simulink model "MGDC_COMPARACION"  (R2025b)
settings: Solver=VariableStepAuto  StartTime=0.0  StopTime=12  RelTol=1e-3
libraries: spsGroundLib x16, spsSeriesRLCBranchLib x7, spsControlledVoltageSourceLib x6, spsCurrentMeasurementLib x6, spsVoltageMeasurementLib x6, slpidlib x3, spsParallelRLCBranchLib x3, spsBreakerLib x2, sps_lib x1
(part 1 of 4)
settings Model: Creator=joseA  LastModifiedBy=joseA

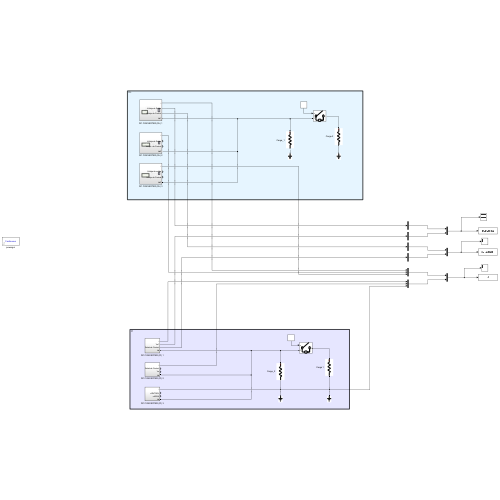
[thumbnail: Simulink's stored preview of the top-level diagram]
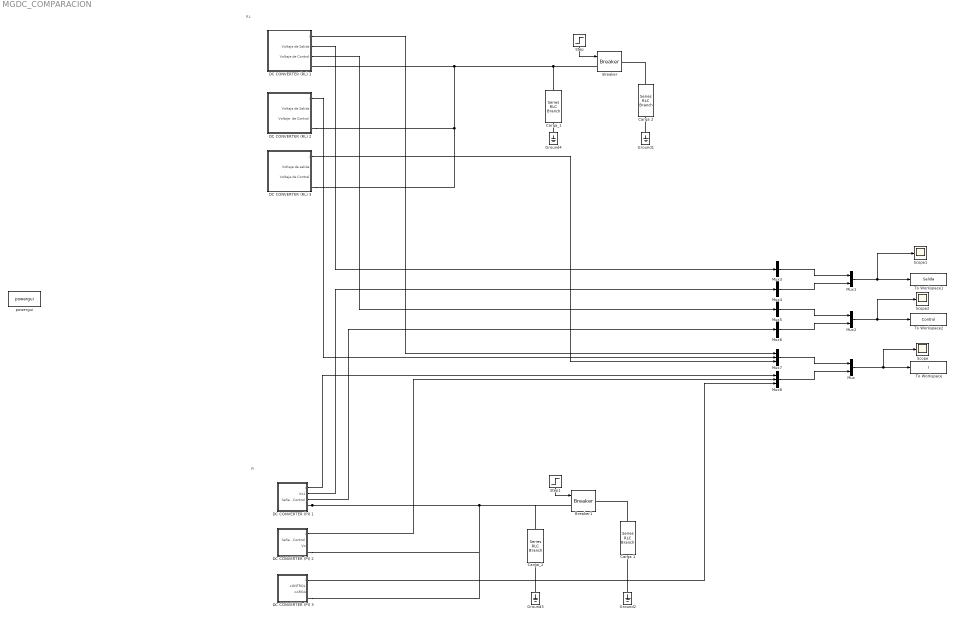
== system MGDC_COMPARACION ==
  note: RL
  note: PI
  Breaker : spsBreakerLib/Breaker  InitialState=0  SwitchingTimes="[1/60  5/60]"  External=on  BreakerResistance=0.01  SnubberResistance=1e6  SnubberCapacitance=inf  Measurements=None  MoreParameters=on  NoBreakLoop=off
  Breaker1 : spsBreakerLib/Breaker  InitialState=0  SwitchingTimes="[1/60  5/60]"  External=on  BreakerResistance=0.01  SnubberResistance=1e6  SnubberCapacitance=inf  Measurements=None  MoreParameters=on  NoBreakLoop=off
  Carga 1 : spsSeriesRLCBranchLib/Series RLC Branch  LConnTagsString=__new0  RConnTagsString=__new0  BranchType=R  Resistance=4  Inductance=1e-3  SetiL0=off  InitialCurrent=0  Capacitance=1e-6  Setx0=off  InitialVoltage=0  Measurements=None
  Carga 2 : spsSeriesRLCBranchLib/Series RLC Branch  LConnTagsString=__new0  RConnTagsString=__new0  BranchType=R  Resistance=4  Inductance=1e-3  SetiL0=off  InitialCurrent=0  Capacitance=1e-6  Setx0=off  InitialVoltage=0  Measurements=None
  Carga_1 : spsSeriesRLCBranchLib/Series RLC Branch  LConnTagsString=__new0  RConnTagsString=__new0  BranchType=R  Resistance=8  Inductance=1e-3  SetiL0=off  InitialCurrent=0  Capacitance=1e-6  Setx0=off  InitialVoltage=0  Measurements=None
  Carga_2 : spsSeriesRLCBranchLib/Series RLC Branch  LConnTagsString=__new0  RConnTagsString=__new0  BranchType=R  Resistance=8  Inductance=1e-3  SetiL0=off  InitialCurrent=0  Capacitance=1e-6  Setx0=off  InitialVoltage=0  Measurements=None
  DC CONVERTER (PI) 1 : Subsystem
      settings: PortSchema="{\"entries\":[{\"content\":{\"sides\":[{\"content\":{\"connectorIds\":[\"Out1\",\"Out2\",\"Out3\",\"LConn1\"]},\"type\":\"ConnectorPlacement.EquallySpacedRectSide\",\"uuid\":\"35976870-9b6d-41fa-84c3-6a07a84f2598\"},{\"content\":{\"side\":\"RIGHT\"},\"type\":\"ConnectorPlacement.EquallySpacedRectSide\",\"uuid\":\"2aca6fb9-572f-479a-9834-ebae41799751\"},{\"content\":{\"side\":\"TOP\"},\"type\":\"ConnectorPlacement.EquallySpacedRectSide\",\"uuid\":\"9763f1a6-ce88-4779-87cd-07f32833b3c9\"}]},\"type\":\"ConnectorPlacement.EquallySpacedConnector\",\"uuid\":\"787491d0-6cf4-4606-8410-63a22802da97\"}],\"packageUris\":[\"http://schema.mathworks.com/mf0/Connector/R2020b\"],\"version\":\"1.0\"}"
  DC CONVERTER (PI) 2 : Subsystem
      settings: PortSchema="{\"entries\":[{\"content\":{\"sides\":[{\"content\":{\"connectorIds\":[\"Out1\",\"Out2\",\"Out3\",\"LConn1\"]},\"type\":\"ConnectorPlacement.EquallySpacedRectSide\",\"uuid\":\"35976870-9b6d-41fa-84c3-6a07a84f2598\"},{\"content\":{\"side\":\"RIGHT\"},\"type\":\"ConnectorPlacement.EquallySpacedRectSide\",\"uuid\":\"2aca6fb9-572f-479a-9834-ebae41799751\"},{\"content\":{\"side\":\"TOP\"},\"type\":\"ConnectorPlacement.EquallySpacedRectSide\",\"uuid\":\"9763f1a6-ce88-4779-87cd-07f32833b3c9\"}]},\"type\":\"ConnectorPlacement.EquallySpacedConnector\",\"uuid\":\"787491d0-6cf4-4606-8410-63a22802da97\"}],\"packageUris\":[\"http://schema.mathworks.com/mf0/Connector/R2020b\"],\"version\":\"1.0\"}"
  DC CONVERTER (PI) 3 : Subsystem
      settings: PortSchema="{\"entries\":[{\"content\":{\"sides\":[{\"content\":{\"connectorIds\":[\"Out1\",\"Out2\",\"Out3\",\"LConn1\"]},\"type\":\"ConnectorPlacement.EquallySpacedRectSide\",\"uuid\":\"35976870-9b6d-41fa-84c3-6a07a84f2598\"},{\"content\":{\"side\":\"RIGHT\"},\"type\":\"ConnectorPlacement.EquallySpacedRectSide\",\"uuid\":\"2aca6fb9-572f-479a-9834-ebae41799751\"},{\"content\":{\"side\":\"TOP\"},\"type\":\"ConnectorPlacement.EquallySpacedRectSide\",\"uuid\":\"9763f1a6-ce88-4779-87cd-07f32833b3c9\"}]},\"type\":\"ConnectorPlacement.EquallySpacedConnector\",\"uuid\":\"787491d0-6cf4-4606-8410-63a22802da97\"}],\"packageUris\":[\"http://schema.mathworks.com/mf0/Connector/R2020b\"],\"version\":\"1.0\"}"
  DC CONVERTER (RL) 1 : Subsystem
      settings: PortSchema="{\"entries\":[{\"content\":{\"sides\":[{\"content\":{\"connectorIds\":[\"Out1\",\"Out2\",\"Out3\",\"LConn1\"]},\"type\":\"ConnectorPlacement.EquallySpacedRectSide\",\"uuid\":\"ef85fad9-e9fc-446c-84f1-0628c69dc682\"},{\"content\":{\"side\":\"RIGHT\"},\"type\":\"ConnectorPlacement.EquallySpacedRectSide\",\"uuid\":\"b40e7fcd-3dee-4863-8a64-1e7c5a18af7f\"},{\"content\":{\"side\":\"TOP\"},\"type\":\"ConnectorPlacement.EquallySpacedRectSide\",\"uuid\":\"d80d7a5f-fa61-4dc2-bf12-1a6ce1f92f0b\"}]},\"type\":\"ConnectorPlacement.EquallySpacedConnector\",\"uuid\":\"ea08e065-469c-42e9-9976-17e3ee08db16\"}],\"packageUris\":[\"http://schema.mathworks.com/mf0/Connector/R2020b\"],\"version\":\"1.0\"}"
  DC CONVERTER (RL) 2 : Subsystem
      settings: PortSchema="{\"entries\":[{\"content\":{\"sides\":[{\"content\":{\"connectorIds\":[\"Out1\",\"Out2\",\"Out3\",\"LConn1\"]},\"type\":\"ConnectorPlacement.EquallySpacedRectSide\",\"uuid\":\"ef85fad9-e9fc-446c-84f1-0628c69dc682\"},{\"content\":{\"side\":\"RIGHT\"},\"type\":\"ConnectorPlacement.EquallySpacedRectSide\",\"uuid\":\"b40e7fcd-3dee-4863-8a64-1e7c5a18af7f\"},{\"content\":{\"side\":\"TOP\"},\"type\":\"ConnectorPlacement.EquallySpacedRectSide\",\"uuid\":\"d80d7a5f-fa61-4dc2-bf12-1a6ce1f92f0b\"}]},\"type\":\"ConnectorPlacement.EquallySpacedConnector\",\"uuid\":\"ea08e065-469c-42e9-9976-17e3ee08db16\"}],\"packageUris\":[\"http://schema.mathworks.com/mf0/Connector/R2020b\"],\"version\":\"1.0\"}"
  DC CONVERTER (RL) 3 : Subsystem
      settings: PortSchema="{\"entries\":[{\"content\":{\"sides\":[{\"content\":{\"connectorIds\":[\"Out1\",\"Out2\",\"Out3\",\"LConn1\"]},\"type\":\"ConnectorPlacement.EquallySpacedRectSide\",\"uuid\":\"ef85fad9-e9fc-446c-84f1-0628c69dc682\"},{\"content\":{\"side\":\"RIGHT\"},\"type\":\"ConnectorPlacement.EquallySpacedRectSide\",\"uuid\":\"b40e7fcd-3dee-4863-8a64-1e7c5a18af7f\"},{\"content\":{\"side\":\"TOP\"},\"type\":\"ConnectorPlacement.EquallySpacedRectSide\",\"uuid\":\"d80d7a5f-fa61-4dc2-bf12-1a6ce1f92f0b\"}]},\"type\":\"ConnectorPlacement.EquallySpacedConnector\",\"uuid\":\"ea08e065-469c-42e9-9976-17e3ee08db16\"}],\"packageUris\":[\"http://schema.mathworks.com/mf0/Connector/R2020b\"],\"version\":\"1.0\"}"
  Ground{1..4} (4 alike) : spsGroundLib/Ground  LConnTagsString=a
  Mux : Mux  Inputs=2
  Mux1 : Mux  Inputs=2
  Mux2 : Mux  Inputs=2
  Mux{3..6} (4 alike) : Mux  Inputs=1
  Mux7 : Mux  Inputs=3
  Mux8 : Mux  Inputs=3
  Scope : Scope
      settings: ActiveDisplayYMinimum=-0.45527999273700881  ActiveDisplayYMaximum=4.74994391053149
  Scope1 : Scope
      settings: ActiveDisplayYMinimum=21.795935750117668  ActiveDisplayYMaximum=24.098400490338538  DataLoggingVariableName=ScopeData4
  Scope2 : Scope
      settings: ActiveDisplayYMinimum=-3.0400673086386818  ActiveDisplayYMaximum=27.410605777748142  DataLoggingVariableName=ScopeData2
  Step : Step  Time=6.5  SampleTime=0
  Step1 : Step  Time=6.5  SampleTime=0
  To Workspace : ToWorkspace  VariableName=I  SaveFormat=Timeseries  SampleTime=-1
  To Workspace1 : ToWorkspace  VariableName=Salida  SaveFormat=Timeseries  SampleTime=-1
  To Workspace2 : ToWorkspace  VariableName=Control  SaveFormat=Timeseries  SampleTime=-1
  powergui : sps_lib/powergui  Priority=1  SimulationMode=Continuous  SampleTime=50e-6  frequency=60  Iterations=50  frequencyindice=0  Pbase=100e6  ErrMax=1e-4  UnitsV=kV  UnitsW=MW  buscounter=0  FunctionMessages=off  echomessages=off  EnableUseOfTLC=off  CurrentSourceSwitches=off  DisableSnubberDevices=off  DisableRonSwitches=off  DisableVfSwitches=off  DisplayEquations=off  AutomaticDiscreteSolvers=off  SolverType=Tustin/Backward Euler (TBE)  Interpol=off  ExternalGateDelay=off  methode=off  Ts=100  x0status=blocks  SPID=on  SwTol=0  HookPort=off  NonlinearTolerance=1e-4  nMaxIteration=100  ContinueOnMaxIteration=off  RestoreLinks=warning  ResistiveCurrentMeasurement=off  Frange=[0:2:500]  Ylog=off  Xlog=on  ShowGrid=off  save=off  variable=ZData  structure=0  ZoomFFT=off  StartTime=0.0  cycles=1  DisplayStyle=1  fundamental=60  FreqAxis=off  MaxFrequency=1000  frequencyindicesteady=1  RmsSteady=1  display=off
  wires:
  DC CONVERTER (PI) 1/3(Señal de Control) -> Mux6/1
  DC CONVERTER (PI) 1/1(i) -> Mux8/1
  Mux5/1 -> Mux2/1
  Mux7/1 -> Mux/1
  Mux3/1 -> Mux1/1
  DC CONVERTER (PI) 1/2(Vo1) -> Mux4/1
  Mux4/1 -> Mux1/2
  DC CONVERTER (PI) 2/1(i) -> Mux8/2
  Mux6/1 -> Mux2/2
  DC CONVERTER (RL) 1/3(Voltaje de Control) -> Mux5/1
  DC CONVERTER (RL) 1/1(i) -> Mux7/1
  DC CONVERTER (RL) 1/2(Voltaje de Salida) -> Mux3/1
  Mux2/1 -> Scope2/1, To Workspace2/1
  Step/1 -> Breaker/1
  Mux/1 -> To Workspace/1, Scope/1
  DC CONVERTER (PI) 3/1(i) -> Mux8/3
  Mux8/1 -> Mux/2
  Mux1/1 -> To Workspace1/1, Scope1/1
  DC CONVERTER (RL) 3/1(i) -> Mux7/3
  Step1/1 -> Breaker1/1
  DC CONVERTER (RL) 2/1(i) -> Mux7/2
  connections:
  DC CONVERTER (PI) 1/LConn1 -- Breaker1/LConn1 -- Carga_2/LConn1 -- DC CONVERTER (PI) 3/LConn1 -- DC CONVERTER (PI) 2/LConn1
  DC CONVERTER (RL) 3/LConn1 -- DC CONVERTER (RL) 2/LConn1 -- Breaker/LConn1 -- Carga_1/LConn1 -- DC CONVERTER (RL) 1/LConn1
  Carga 1/LConn1 -- Breaker1/RConn1
  Ground1/LConn1 -- Carga 2/RConn1
  Ground3/LConn1 -- Carga_2/RConn1
  Ground2/LConn1 -- Carga 1/RConn1
  Ground4/LConn1 -- Carga_1/RConn1
  Carga 2/LConn1 -- Breaker/RConn1

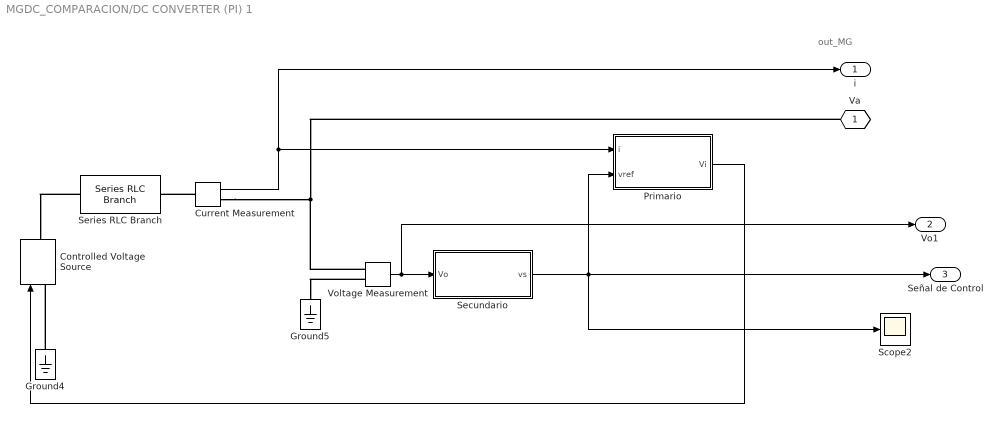
== system MGDC_COMPARACION/DC CONVERTER (PI) 1 ==
  note: out_MG
  Controlled Voltage Source : spsControlledVoltageSourceLib/Controlled Voltage Source  Initialize=on  Source_Type=DC  Amplitude=0  Phase=0  Frequency=0  Measurements=None
  Current Measurement : spsCurrentMeasurementLib/Current Measurement  PhasorSimulation=off  OutputType=Complex  PSBequivalent=0
  Ground4 : spsGroundLib/Ground  LConnTagsString=a
  Ground5 : spsGroundLib/Ground  LConnTagsString=a
  Primario : Subsystem
  Scope2 : Scope
      settings: ActiveDisplayYMinimum=21.641164987150439  ActiveDisplayYMaximum=24.237473255707151  DataLoggingVariableName=ScopeData3
  Secundario : Subsystem
  Series RLC Branch : spsSeriesRLCBranchLib/Series RLC Branch  LConnTagsString=__new0  RConnTagsString=__new0  BranchType=R  Resistance=0.1  Inductance=1e-3  SetiL0=off  InitialCurrent=0  Capacitance=1e-6  Setx0=off  InitialVoltage=0  Measurements=None
  Voltage Measurement : spsVoltageMeasurementLib/Voltage Measurement  PhasorSimulation=off  OutputType=Complex  PSBequivalent=0
  Va : PMIOPort  Tag=PMCPort  Side=Left
  i : Outport
  Vo1 : Outport  Port=2
  Señal de Control : Outport  Port=3
  wires:
  Voltage Measurement/1 -> Vo1/1, Secundario/1(Vo)
  Current Measurement/1 -> i/1, Primario/1(i)
  Secundario/1(vs) -> Primario/2(vref), Señal de Control/1, Scope2/1
  Primario/1(Vi) -> Controlled Voltage Source/1
  connections:
  Series RLC Branch/LConn1 -- Controlled Voltage Source/RConn1
  Ground4/LConn1 -- Controlled Voltage Source/LConn1
  Current Measurement/LConn1 -- Series RLC Branch/RConn1
  Current Measurement/RConn1 -- Voltage Measurement/LConn1 -- Va/RConn1
  Voltage Measurement/LConn2 -- Ground5/LConn1

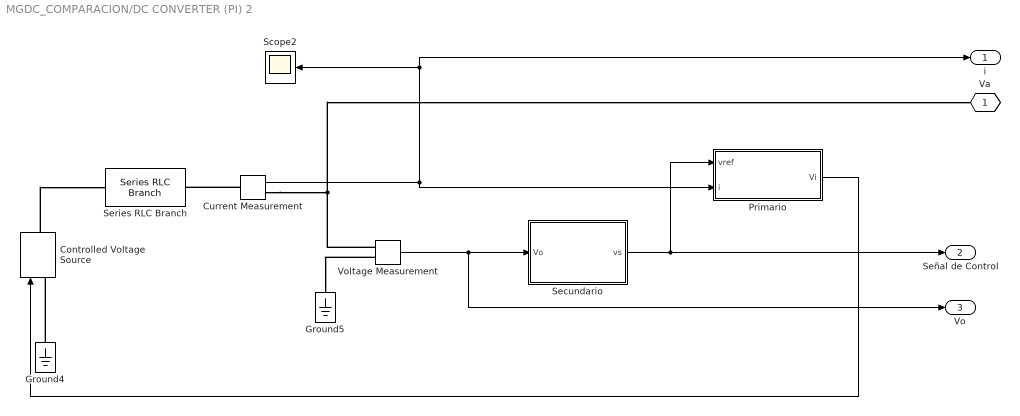
== system MGDC_COMPARACION/DC CONVERTER (PI) 2 ==
  Controlled Voltage Source : spsControlledVoltageSourceLib/Controlled Voltage Source  Initialize=on  Source_Type=DC  Amplitude=0  Phase=0  Frequency=0  Measurements=None
  Current Measurement : spsCurrentMeasurementLib/Current Measurement  PhasorSimulation=off  OutputType=Complex  PSBequivalent=0
  Ground4 : spsGroundLib/Ground  LConnTagsString=a
  Ground5 : spsGroundLib/Ground  LConnTagsString=a
  Primario : Subsystem
  Scope2 : Scope
      settings: ActiveDisplayYMinimum=26.65957  ActiveDisplayYMaximum=30.33414
  Secundario : Subsystem
  Series RLC Branch : spsSeriesRLCBranchLib/Series RLC Branch  LConnTagsString=__new0  RConnTagsString=__new0  BranchType=R  Resistance=0.1  Inductance=1e-3  SetiL0=off  InitialCurrent=0  Capacitance=1e-6  Setx0=off  InitialVoltage=0  Measurements=None
  Voltage Measurement : spsVoltageMeasurementLib/Voltage Measurement  PhasorSimulation=off  OutputType=Complex  PSBequivalent=0
  Va : PMIOPort  Tag=PMCPort  Side=Left
  i : Outport
  Señal de Control : Outport  Port=2
  Vo : Outport  Port=3
  wires:
  Primario/1(Vi) -> Controlled Voltage Source/1
  Secundario/1(vs) -> Primario/1(vref), Señal de Control/1
  Current Measurement/1 -> i/1, Scope2/1, Primario/2(i)
  Voltage Measurement/1 -> Vo/1, Secundario/1(Vo)
  connections:
  Voltage Measurement/LConn2 -- Ground5/LConn1
  Voltage Measurement/LConn1 -- Va/RConn1 -- Current Measurement/RConn1
  Current Measurement/LConn1 -- Series RLC Branch/RConn1
  Ground4/LConn1 -- Controlled Voltage Source/LConn1
  Controlled Voltage Source/RConn1 -- Series RLC Branch/LConn1

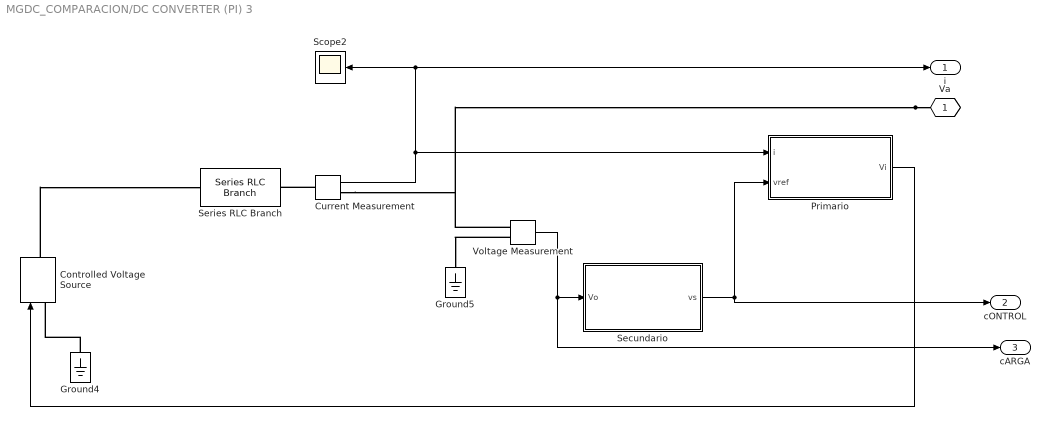
== system MGDC_COMPARACION/DC CONVERTER (PI) 3 ==
  Controlled Voltage Source : spsControlledVoltageSourceLib/Controlled Voltage Source  Initialize=on  Source_Type=DC  Amplitude=0  Phase=0  Frequency=0  Measurements=None
  Current Measurement : spsCurrentMeasurementLib/Current Measurement  PhasorSimulation=off  OutputType=Complex  PSBequivalent=0
  Ground4 : spsGroundLib/Ground  LConnTagsString=a
  Ground5 : spsGroundLib/Ground  LConnTagsString=a
  Primario : Subsystem
  Scope2 : Scope
      settings: ActiveDisplayYMinimum=-2.79721  ActiveDisplayYMaximum=25.17493
  Secundario : Subsystem
  Series RLC Branch : spsSeriesRLCBranchLib/Series RLC Branch  LConnTagsString=__new0  RConnTagsString=__new0  BranchType=R  Resistance=0.1  Inductance=1e-3  SetiL0=off  InitialCurrent=0  Capacitance=1e-6  Setx0=off  InitialVoltage=0  Measurements=None
  Voltage Measurement : spsVoltageMeasurementLib/Voltage Measurement  PhasorSimulation=off  OutputType=Complex  PSBequivalent=0
  Va : PMIOPort  Tag=PMCPort  Side=Left
  i : Outport
  cONTROL : Outport  Port=2
  cARGA : Outport  Port=3
  wires:
  Primario/1(Vi) -> Controlled Voltage Source/1
  Secundario/1(vs) -> cONTROL/1, Primario/2(vref)
  Current Measurement/1 -> i/1, Scope2/1, Primario/1(i)
  Voltage Measurement/1 -> cARGA/1, Secundario/1(Vo)
  connections:
  Controlled Voltage Source/RConn1 -- Series RLC Branch/LConn1
  Voltage Measurement/LConn2 -- Ground5/LConn1
  Va/RConn1 -- Voltage Measurement/LConn1 -- Current Measurement/RConn1
  Current Measurement/LConn1 -- Series RLC Branch/RConn1
  Ground4/LConn1 -- Controlled Voltage Source/LConn1

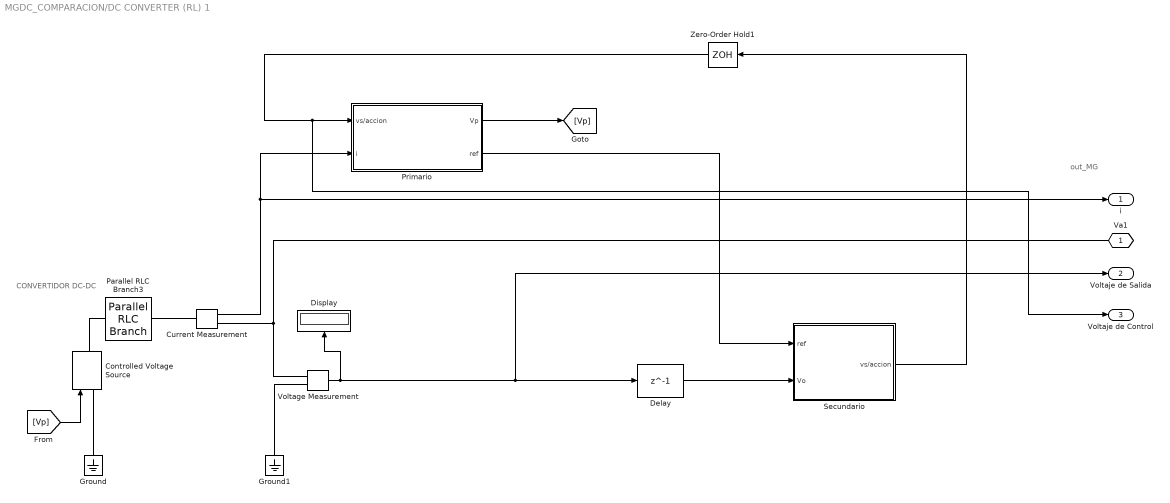
== system MGDC_COMPARACION/DC CONVERTER (RL) 1 ==
  note: out_MG
  note: CONVERTIDOR DC-DC
  Controlled Voltage Source : spsControlledVoltageSourceLib/Controlled Voltage Source  Initialize=on  Source_Type=DC  Amplitude=0  Phase=0  Frequency=0  Measurements=None
  Current Measurement : spsCurrentMeasurementLib/Current Measurement  PhasorSimulation=off  OutputType=Complex  PSBequivalent=0
  Delay : Delay  DelayLength=1  InitialCondition=0  UseCircularBuffer=on
  Display : Display
  Ground : spsGroundLib/Ground  LConnTagsString=a
  Ground1 : spsGroundLib/Ground  LConnTagsString=a
  Parallel RLC Branch3 : spsParallelRLCBranchLib/Parallel RLC Branch  LConnTagsString=a  RConnTagsString=__new0  BranchType=R  Resistance=0.01  Inductance=1e-3  SetiL0=off  InitialCurrent=0  Capacitance=1e-6  Setx0=off  InitialVoltage=0  Measurements=None
  Primario : Subsystem
  "Secundario " : Subsystem
  Voltage Measurement : spsVoltageMeasurementLib/Voltage Measurement  PhasorSimulation=off  OutputType=Complex  PSBequivalent=0
  Zero-Order Hold1 : ZeroOrderHold  SampleTime=0.01
  Va1 : PMIOPort  Tag=PMCPort  Side=Left
  i : Outport
  Voltaje de Salida : Outport  Port=2
  Voltaje de Control : Outport  Port=3
  wires:
  Voltage Measurement/1 -> Voltaje de Salida/1, Delay/1, Display/1
  [Vp] -> Controlled Voltage Source/1
  Zero-Order Hold1/1 -> Voltaje de Control/1, Primario/1(vs/accion)
  Current Measurement/1 -> i/1, Primario/2(i)
  "Secundario "/1(vs/accion) -> Zero-Order Hold1/1
  Primario/2(ref) -> "Secundario "/1(ref)
  Delay/1 -> "Secundario "/2(Vo)
  Primario/1(Vp) -> [Vp]
  connections:
  Voltage Measurement/LConn2 -- Ground1/LConn1
  Ground/LConn1 -- Controlled Voltage Source/LConn1
  Parallel RLC Branch3/LConn1 -- Current Measurement/LConn1
  Voltage Measurement/LConn1 -- Va1/RConn1 -- Current Measurement/RConn1
  Controlled Voltage Source/RConn1 -- Parallel RLC Branch3/RConn1

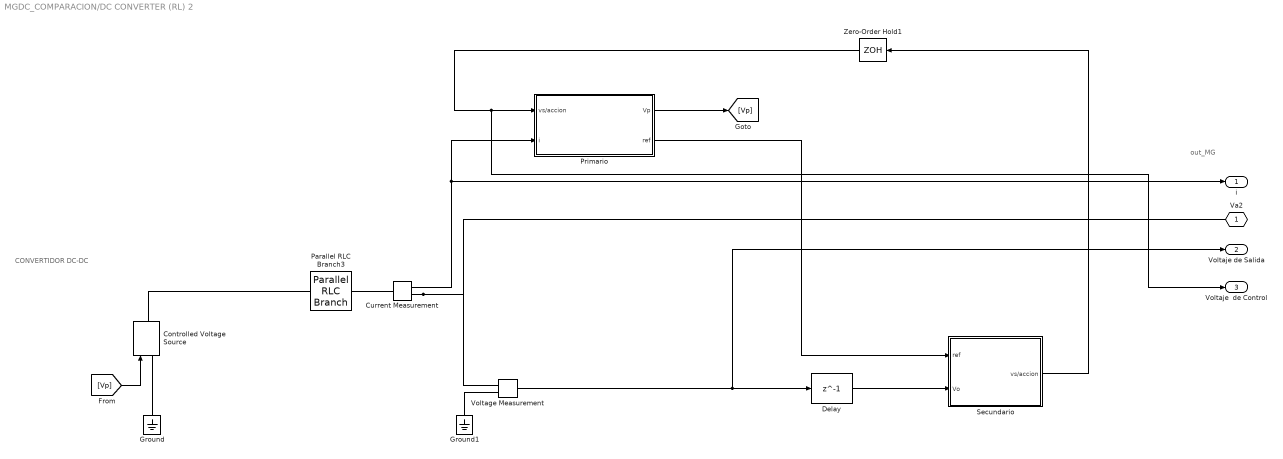
== system MGDC_COMPARACION/DC CONVERTER (RL) 2 ==
  note: out_MG
  note: CONVERTIDOR DC-DC
  Controlled Voltage Source : spsControlledVoltageSourceLib/Controlled Voltage Source  Initialize=on  Source_Type=DC  Amplitude=0  Phase=0  Frequency=0  Measurements=None
  Current Measurement : spsCurrentMeasurementLib/Current Measurement  PhasorSimulation=off  OutputType=Complex  PSBequivalent=0
  Delay : Delay  DelayLength=1  InitialCondition=0  UseCircularBuffer=on
  Ground : spsGroundLib/Ground  LConnTagsString=a
  Ground1 : spsGroundLib/Ground  LConnTagsString=a
  Parallel RLC Branch3 : spsParallelRLCBranchLib/Parallel RLC Branch  LConnTagsString=a  RConnTagsString=__new0  BranchType=R  Resistance=0.01  Inductance=1e-3  SetiL0=off  InitialCurrent=0  Capacitance=1e-6  Setx0=off  InitialVoltage=0  Measurements=None
  Primario : Subsystem
  "Secundario " : Subsystem
  Voltage Measurement : spsVoltageMeasurementLib/Voltage Measurement  PhasorSimulation=off  OutputType=Complex  PSBequivalent=0
  Zero-Order Hold1 : ZeroOrderHold  SampleTime=0.01
  Va2 : PMIOPort  Tag=PMCPort  Side=Left
  i : Outport
  Voltaje de Salida : Outport  Port=2
  Voltaje  de Control : Outport  Port=3
  wires:
  Voltage Measurement/1 -> Voltaje de Salida/1, Delay/1
  [Vp] -> Controlled Voltage Source/1
  Zero-Order Hold1/1 -> Voltaje  de Control/1, Primario/1(vs/accion)
  Current Measurement/1 -> i/1, Primario/2(i)
  "Secundario "/1(vs/accion) -> Zero-Order Hold1/1
  Primario/2(ref) -> "Secundario "/1(ref)
  Primario/1(Vp) -> [Vp]
  Delay/1 -> "Secundario "/2(Vo)
  connections:
  Voltage Measurement/LConn2 -- Ground1/LConn1
  Ground/LConn1 -- Controlled Voltage Source/LConn1
  Current Measurement/LConn1 -- Parallel RLC Branch3/LConn1
  Current Measurement/RConn1 -- Voltage Measurement/LConn1 -- Va2/RConn1
  Controlled Voltage Source/RConn1 -- Parallel RLC Branch3/RConn1

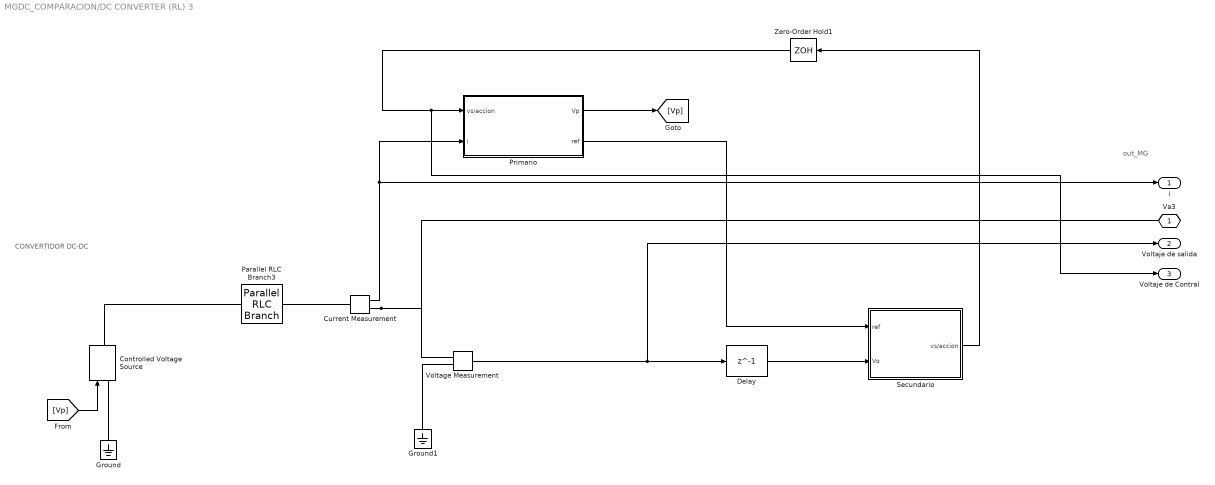
== system MGDC_COMPARACION/DC CONVERTER (RL) 3 ==
  note: out_MG
  note: CONVERTIDOR DC-DC
  Controlled Voltage Source : spsControlledVoltageSourceLib/Controlled Voltage Source  Initialize=on  Source_Type=DC  Amplitude=0  Phase=0  Frequency=0  Measurements=None
  Current Measurement : spsCurrentMeasurementLib/Current Measurement  PhasorSimulation=off  OutputType=Complex  PSBequivalent=0
  Delay : Delay  DelayLength=1  InitialCondition=0  UseCircularBuffer=on
  Ground : spsGroundLib/Ground  LConnTagsString=a
  Ground1 : spsGroundLib/Ground  LConnTagsString=a
  Parallel RLC Branch3 : spsParallelRLCBranchLib/Parallel RLC Branch  LConnTagsString=a  RConnTagsString=__new0  BranchType=R  Resistance=0.01  Inductance=1e-3  SetiL0=off  InitialCurrent=0  Capacitance=1e-6  Setx0=off  InitialVoltage=0  Measurements=None
  Primario : Subsystem
  "Secundario " : Subsystem
  Voltage Measurement : spsVoltageMeasurementLib/Voltage Measurement  PhasorSimulation=off  OutputType=Complex  PSBequivalent=0
  Zero-Order Hold1 : ZeroOrderHold  SampleTime=0.01
  Va3 : PMIOPort  Tag=PMCPort  Side=Left
  i : Outport
  Voltaje de salida : Outport  Port=2
  Voltaje de Contral : Outport  Port=3
  wires:
  Voltage Measurement/1 -> Voltaje de salida/1, Delay/1
  [Vp] -> Controlled Voltage Source/1
  Zero-Order Hold1/1 -> Voltaje de Contral/1, Primario/1(vs/accion)
  Current Measurement/1 -> i/1, Primario/2(i)
  "Secundario "/1(vs/accion) -> Zero-Order Hold1/1
  Primario/2(ref) -> "Secundario "/1(ref)
  Delay/1 -> "Secundario "/2(Vo)
  Primario/1(Vp) -> [Vp]
  connections:
  Voltage Measurement/LConn2 -- Ground1/LConn1
  Ground/LConn1 -- Controlled Voltage Source/LConn1
  Current Measurement/LConn1 -- Parallel RLC Branch3/LConn1
  Current Measurement/RConn1 -- Voltage Measurement/LConn1 -- Va3/RConn1
  Controlled Voltage Source/RConn1 -- Parallel RLC Branch3/RConn1

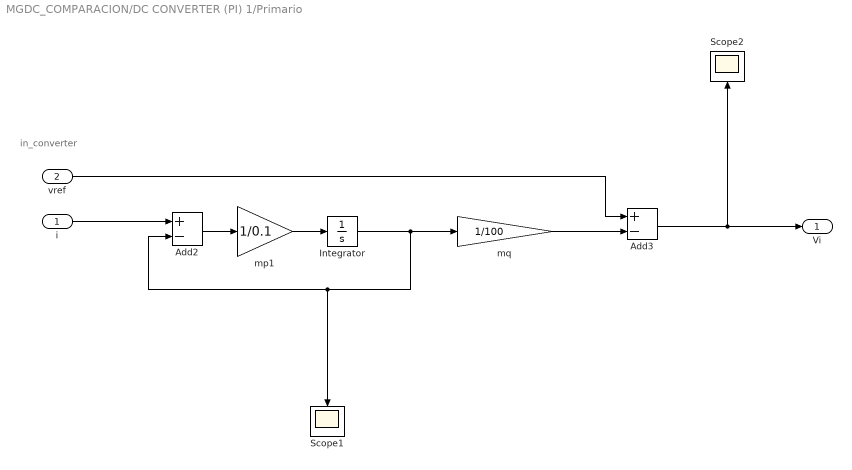
== system MGDC_COMPARACION/DC CONVERTER (PI) 1/Primario ==
  note: in_converter
  i : Inport
  vref : Inport  Port=2
  Add2 : Sum  Inputs=+-
  Add3 : Sum  Inputs=+-
  Integrator : Integrator
  Scope1 : Scope
      settings: ActiveDisplayYMinimum=-1.73796  ActiveDisplayYMaximum=15.64167  DataLoggingVariableName=ScopeData10
  Scope2 : Scope
      settings: ActiveDisplayYMinimum=21.645925037020149  ActiveDisplayYMaximum=24.667369537836731  DataLoggingVariableName=ScopeData11
  mp1 : Gain  Gain=1/0.1
  mq : Gain  Gain=1/100
  Vi : Outport
  wires:
  Add2/1 -> mp1/1
  Integrator/1 -> mq/1, Add2/2, Scope1/1
  mp1/1 -> Integrator/1
  mq/1 -> Add3/2
  i/1 -> Add2/1
  vref/1 -> Add3/1
  Add3/1 -> Vi/1, Scope2/1

== system MGDC_COMPARACION/DC CONVERTER (PI) 1/Secundario ==
  Vo : Inport
  Add3 : Sum  Inputs=+-
  PID Controller : slpidlib/PID Controller  Controller=PI  Form=Parallel  TimeDomain=Continuous-time  UseExternalTs=off  SampleTime=-1  IntegratorMethod=Forward Euler  FilterMethod=Forward Euler  ControllerParametersSource=internal  P=10  I=10  UseKiTs=off  D=0  UseExternalDerivativeSource=off  N=100  UseFilter=on  TunerSelectOption=Transfer Function Based (PID Tuner App)  InitialConditionSource=internal  InitialConditionForIntegrator=0  InitialConditionForFilter=0  DifferentiatorICPrevScaledInput=0  ExternalReset=none  TrackingMode=off  Kt=1  LimitOutput=off  SatLimitsSource=internal  UpperSaturationLimit=inf  LowerSaturationLimit=-inf  LinearizeAsGain=on  AntiWindupMode=none  Kb=1  LimitIntegrator=off  UpperIntegratorSaturationLimit=inf  LowerIntegratorSaturationLimit=-inf  POutMin=[]  POutMax=[]  IOutMin=[]  IOutMax=[]  DOutMin=[]  DOutMax=[]  NOutMin=[]  NOutMax=[]  SumOutMin=[]  SumOutMax=[]  SaturationOutMin=[]  SaturationOutMax=[]  PParamMin=[]  PParamMax=[]  IParamMin=[]  IParamMax=[]  DParamMin=[]  DParamMax=[]  NParamMin=[]  NParamMax=[]  KbParamMin=[]  KbParamMax=[]  KtParamMin=[]  KtParamMax=[]  KbOutMin=[]  KbOutMax=[]  KtOutMin=[]  KtOutMax=[]  IntegratorOutMin=[]  IntegratorOutMax=[]  FilterOutMin=[]  FilterOutMax=[]  SumI1OutMin=[]  SumI1OutMax=[]  SumI2OutMin=[]  SumI2OutMax=[]  SumI3OutMin=[]  SumI3OutMax=[]  SumI4OutMin=[]  SumI4OutMax=[]  SumDOutMin=[]  SumDOutMax=[]  DifferentiatorOutMin=[]  DifferentiatorOutMax=[]  FilterDiffOutCoefMin=[]  FilterDiffOutCoefMax=[]  ReciprocalOutMin=[]  ReciprocalOutMax=[]  SumDenOutMin=[]  SumDenOutMax=[]  SumNumOutMin=[]  SumNumOutMax=[]  DivideOutMin=[]  DivideOutMax=[]  UdiffTsProdOutMin=[]  UdiffTsProdOutMax=[]  NTsProdOutMin=[]  NTsProdOutMax=[]  UintegralTsProdOutMin=[]  UintegralTsProdOutMax=[]  UngainTsProdOutMin=[]  UngainTsProdOutMax=[]  ClampingZeroOutDataTypeStr=Inherit: Inherit via back propagation  ClampingZeroOutMin=[]  ClampingZeroOutMax=[]  FilterDenConstantOutDataTypeStr=Inherit: Inherit via back propagation  FilterDenConstantOutMin=[]  FilterDenConstantOutMax=[]  PCopyOutDataTypeStr=Inherit: Inherit via back propagation  PCopyOutMin=[]  PCopyOutMax=[]  NCopyOutDataTypeStr=Inherit: Inherit via back propagation  NCopyOutMin=[]  NCopyOutMax=[]  IntegratorContinuousStateAttributes=''  IntegratorStateMustResolveToSignalObject=off  IntegratorRTWStateStorageClass=Auto  FilterContinuousStateAttributes=''  FilterStateMustResolveToSignalObject=off  FilterRTWStateStorageClass=Auto  ParallelPVariant=InternalParameters  IdealPVariant=Disabled  IVariant=InternalParameters  DVariant=Disabled  IntegratorVariant=Continuous  SatVariant=Disabled  AWVariant=Passthrough  PCopyVariant=Disabled  TRVariant=Disabled  FdbkBlocksVariant=Forward  IdealPFdbkVariant=Disabled  SatFdbkVariant=Disabled  DerivativeFilterVariant=Disabled  NVariant=Disabled  NCopyVariant=Disabled_SignalSpec  FilterICVariant=Disabled  IntegratorICVariant=InternalICs  ExternalResetVariant=Disabled  TRSumVariant=Passthrough  SumFdbkVariant=Disabled  SumVariant=Sum_PI  TsampFilterVariant=InternalTs  TsampNgainVariant=Passthrough  TsampIntegralVariant=Disabled_SignalSpec  ExternalSaturationOutDataTypeStr=Inherit: Same as second input  DerivativeSourceVariant=Disabled  PreIntVariant=InternalPreInt
  Vref : Constant  Value=24
  vs : Outport
  wires:
  Vref/1 -> Add3/1
  Add3/1 -> PID Controller/1
  PID Controller/1 -> vs/1
  Vo/1 -> Add3/2

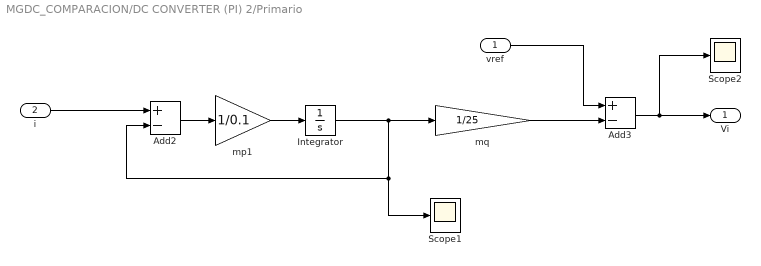
== system MGDC_COMPARACION/DC CONVERTER (PI) 2/Primario ==
  vref : Inport
  i : Inport  Port=2
  Add2 : Sum  Inputs=+-
  Add3 : Sum  Inputs=+-
  Integrator : Integrator
  Scope1 : Scope
      settings: ActiveDisplayYMinimum=-1.781  ActiveDisplayYMaximum=16.02899  DataLoggingVariableName=ScopeData10
  Scope2 : Scope
      settings: ActiveDisplayYMinimum=29.32553  ActiveDisplayYMaximum=33.36756  DataLoggingVariableName=ScopeData11
  mp1 : Gain  Gain=1/0.1
  mq : Gain  Gain=1/25
  Vi : Outport
  wires:
  vref/1 -> Add3/1
  Add3/1 -> Scope2/1, Vi/1
  i/1 -> Add2/1
  mq/1 -> Add3/2
  mp1/1 -> Integrator/1
  Integrator/1 -> Scope1/1, Add2/2, mq/1
  Add2/1 -> mp1/1

== system MGDC_COMPARACION/DC CONVERTER (PI) 2/Secundario ==
  Vo : Inport
  Add3 : Sum  Inputs=+-
  PID Controller : slpidlib/PID Controller  Controller=PI  Form=Parallel  TimeDomain=Continuous-time  UseExternalTs=off  SampleTime=-1  IntegratorMethod=Forward Euler  FilterMethod=Forward Euler  ControllerParametersSource=internal  P=10  I=10  UseKiTs=off  D=0  UseExternalDerivativeSource=off  N=100  UseFilter=on  TunerSelectOption=Transfer Function Based (PID Tuner App)  InitialConditionSource=internal  InitialConditionForIntegrator=0  InitialConditionForFilter=0  DifferentiatorICPrevScaledInput=0  ExternalReset=none  TrackingMode=off  Kt=1  LimitOutput=off  SatLimitsSource=internal  UpperSaturationLimit=inf  LowerSaturationLimit=-inf  LinearizeAsGain=on  AntiWindupMode=none  Kb=1  LimitIntegrator=off  UpperIntegratorSaturationLimit=inf  LowerIntegratorSaturationLimit=-inf  POutMin=[]  POutMax=[]  IOutMin=[]  IOutMax=[]  DOutMin=[]  DOutMax=[]  NOutMin=[]  NOutMax=[]  SumOutMin=[]  SumOutMax=[]  SaturationOutMin=[]  SaturationOutMax=[]  PParamMin=[]  PParamMax=[]  IParamMin=[]  IParamMax=[]  DParamMin=[]  DParamMax=[]  NParamMin=[]  NParamMax=[]  KbParamMin=[]  KbParamMax=[]  KtParamMin=[]  KtParamMax=[]  KbOutMin=[]  KbOutMax=[]  KtOutMin=[]  KtOutMax=[]  IntegratorOutMin=[]  IntegratorOutMax=[]  FilterOutMin=[]  FilterOutMax=[]  SumI1OutMin=[]  SumI1OutMax=[]  SumI2OutMin=[]  SumI2OutMax=[]  SumI3OutMin=[]  SumI3OutMax=[]  SumI4OutMin=[]  SumI4OutMax=[]  SumDOutMin=[]  SumDOutMax=[]  DifferentiatorOutMin=[]  DifferentiatorOutMax=[]  FilterDiffOutCoefMin=[]  FilterDiffOutCoefMax=[]  ReciprocalOutMin=[]  ReciprocalOutMax=[]  SumDenOutMin=[]  SumDenOutMax=[]  SumNumOutMin=[]  SumNumOutMax=[]  DivideOutMin=[]  DivideOutMax=[]  UdiffTsProdOutMin=[]  UdiffTsProdOutMax=[]  NTsProdOutMin=[]  NTsProdOutMax=[]  UintegralTsProdOutMin=[]  UintegralTsProdOutMax=[]  UngainTsProdOutMin=[]  UngainTsProdOutMax=[]  ClampingZeroOutDataTypeStr=Inherit: Inherit via back propagation  ClampingZeroOutMin=[]  ClampingZeroOutMax=[]  FilterDenConstantOutDataTypeStr=Inherit: Inherit via back propagation  FilterDenConstantOutMin=[]  FilterDenConstantOutMax=[]  PCopyOutDataTypeStr=Inherit: Inherit via back propagation  PCopyOutMin=[]  PCopyOutMax=[]  NCopyOutDataTypeStr=Inherit: Inherit via back propagation  NCopyOutMin=[]  NCopyOutMax=[]  IntegratorContinuousStateAttributes=''  IntegratorStateMustResolveToSignalObject=off  IntegratorRTWStateStorageClass=Auto  FilterContinuousStateAttributes=''  FilterStateMustResolveToSignalObject=off  FilterRTWStateStorageClass=Auto  ParallelPVariant=InternalParameters  IdealPVariant=Disabled  IVariant=InternalParameters  DVariant=Disabled  IntegratorVariant=Continuous  SatVariant=Disabled  AWVariant=Passthrough  PCopyVariant=Disabled  TRVariant=Disabled  FdbkBlocksVariant=Forward  IdealPFdbkVariant=Disabled  SatFdbkVariant=Disabled  DerivativeFilterVariant=Disabled  NVariant=Disabled  NCopyVariant=Disabled_SignalSpec  FilterICVariant=Disabled  IntegratorICVariant=InternalICs  ExternalResetVariant=Disabled  TRSumVariant=Passthrough  SumFdbkVariant=Disabled  SumVariant=Sum_PI  TsampFilterVariant=InternalTs  TsampNgainVariant=Passthrough  TsampIntegralVariant=Disabled_SignalSpec  ExternalSaturationOutDataTypeStr=Inherit: Same as second input  DerivativeSourceVariant=Disabled  PreIntVariant=InternalPreInt
  Vref : Constant  Value=24
  vs : Outport
  wires:
  Vo/1 -> Add3/2
  PID Controller/1 -> vs/1
  Add3/1 -> PID Controller/1
  Vref/1 -> Add3/1

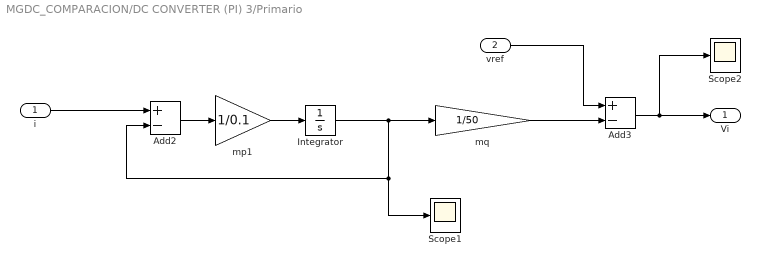
== system MGDC_COMPARACION/DC CONVERTER (PI) 3/Primario ==
  i : Inport
  vref : Inport  Port=2
  Add2 : Sum  Inputs=+-
  Add3 : Sum  Inputs=+-
  Integrator : Integrator
  Scope1 : Scope
      settings: ActiveDisplayYMinimum=-1.33689  ActiveDisplayYMaximum=12.03198  DataLoggingVariableName=ScopeData10
  Scope2 : Scope
      settings: ActiveDisplayYMinimum=29.32553  ActiveDisplayYMaximum=33.36756  DataLoggingVariableName=ScopeData11
  mp1 : Gain  Gain=1/0.1
  mq : Gain  Gain=1/50
  Vi : Outport
  wires:
  vref/1 -> Add3/1
  Add3/1 -> Scope2/1, Vi/1
  i/1 -> Add2/1
  mq/1 -> Add3/2
  mp1/1 -> Integrator/1
  Integrator/1 -> Scope1/1, Add2/2, mq/1
  Add2/1 -> mp1/1

== system MGDC_COMPARACION/DC CONVERTER (PI) 3/Secundario ==
  Vo : Inport
  Add3 : Sum  Inputs=+-
  PID Controller : slpidlib/PID Controller  Controller=PI  Form=Parallel  TimeDomain=Continuous-time  UseExternalTs=off  SampleTime=-1  IntegratorMethod=Forward Euler  FilterMethod=Forward Euler  ControllerParametersSource=internal  P=10  I=10  UseKiTs=off  D=0  UseExternalDerivativeSource=off  N=100  UseFilter=on  TunerSelectOption=Transfer Function Based (PID Tuner App)  InitialConditionSource=internal  InitialConditionForIntegrator=0  InitialConditionForFilter=0  DifferentiatorICPrevScaledInput=0  ExternalReset=none  TrackingMode=off  Kt=1  LimitOutput=off  SatLimitsSource=internal  UpperSaturationLimit=inf  LowerSaturationLimit=-inf  LinearizeAsGain=on  AntiWindupMode=none  Kb=1  LimitIntegrator=off  UpperIntegratorSaturationLimit=inf  LowerIntegratorSaturationLimit=-inf  POutMin=[]  POutMax=[]  IOutMin=[]  IOutMax=[]  DOutMin=[]  DOutMax=[]  NOutMin=[]  NOutMax=[]  SumOutMin=[]  SumOutMax=[]  SaturationOutMin=[]  SaturationOutMax=[]  PParamMin=[]  PParamMax=[]  IParamMin=[]  IParamMax=[]  DParamMin=[]  DParamMax=[]  NParamMin=[]  NParamMax=[]  KbParamMin=[]  KbParamMax=[]  KtParamMin=[]  KtParamMax=[]  KbOutMin=[]  KbOutMax=[]  KtOutMin=[]  KtOutMax=[]  IntegratorOutMin=[]  IntegratorOutMax=[]  FilterOutMin=[]  FilterOutMax=[]  SumI1OutMin=[]  SumI1OutMax=[]  SumI2OutMin=[]  SumI2OutMax=[]  SumI3OutMin=[]  SumI3OutMax=[]  SumI4OutMin=[]  SumI4OutMax=[]  SumDOutMin=[]  SumDOutMax=[]  DifferentiatorOutMin=[]  DifferentiatorOutMax=[]  FilterDiffOutCoefMin=[]  FilterDiffOutCoefMax=[]  ReciprocalOutMin=[]  ReciprocalOutMax=[]  SumDenOutMin=[]  SumDenOutMax=[]  SumNumOutMin=[]  SumNumOutMax=[]  DivideOutMin=[]  DivideOutMax=[]  UdiffTsProdOutMin=[]  UdiffTsProdOutMax=[]  NTsProdOutMin=[]  NTsProdOutMax=[]  UintegralTsProdOutMin=[]  UintegralTsProdOutMax=[]  UngainTsProdOutMin=[]  UngainTsProdOutMax=[]  ClampingZeroOutDataTypeStr=Inherit: Inherit via back propagation  ClampingZeroOutMin=[]  ClampingZeroOutMax=[]  FilterDenConstantOutDataTypeStr=Inherit: Inherit via back propagation  FilterDenConstantOutMin=[]  FilterDenConstantOutMax=[]  PCopyOutDataTypeStr=Inherit: Inherit via back propagation  PCopyOutMin=[]  PCopyOutMax=[]  NCopyOutDataTypeStr=Inherit: Inherit via back propagation  NCopyOutMin=[]  NCopyOutMax=[]  IntegratorContinuousStateAttributes=''  IntegratorStateMustResolveToSignalObject=off  IntegratorRTWStateStorageClass=Auto  FilterContinuousStateAttributes=''  FilterStateMustResolveToSignalObject=off  FilterRTWStateStorageClass=Auto  ParallelPVariant=InternalParameters  IdealPVariant=Disabled  IVariant=InternalParameters  DVariant=Disabled  IntegratorVariant=Continuous  SatVariant=Disabled  AWVariant=Passthrough  PCopyVariant=Disabled  TRVariant=Disabled  FdbkBlocksVariant=Forward  IdealPFdbkVariant=Disabled  SatFdbkVariant=Disabled  DerivativeFilterVariant=Disabled  NVariant=Disabled  NCopyVariant=Disabled_SignalSpec  FilterICVariant=Disabled  IntegratorICVariant=InternalICs  ExternalResetVariant=Disabled  TRSumVariant=Passthrough  SumFdbkVariant=Disabled  SumVariant=Sum_PI  TsampFilterVariant=InternalTs  TsampNgainVariant=Passthrough  TsampIntegralVariant=Disabled_SignalSpec  ExternalSaturationOutDataTypeStr=Inherit: Same as second input  DerivativeSourceVariant=Disabled  PreIntVariant=InternalPreInt
  Vref : Constant  Value=24
  vs : Outport
  wires:
  Vo/1 -> Add3/2
  PID Controller/1 -> vs/1
  Add3/1 -> PID Controller/1
  Vref/1 -> Add3/1

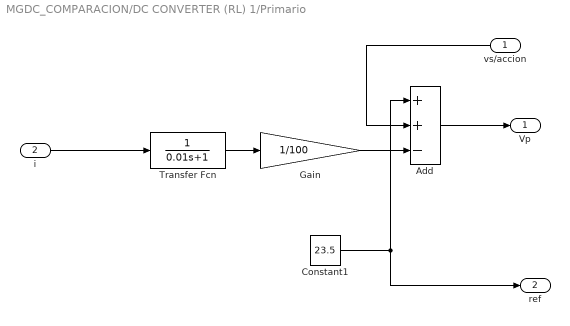
== system MGDC_COMPARACION/DC CONVERTER (RL) 1/Primario ==
  vs/accion : Inport
  i : Inport  Port=2
  Add : Sum  Inputs=++-
  Constant1 : Constant  Value=23.5
  Gain : Gain  Gain=1/100
  Transfer Fcn : TransferFcn  Denominator=[0.01 1]
  Vp : Outport
  ref : Outport  Port=2
  wires:
  vs/accion/1 -> Add/2
  Transfer Fcn/1 -> Gain/1
  Add/1 -> Vp/1
  Constant1/1 -> Add/1, ref/1
  Gain/1 -> Add/3
  i/1 -> Transfer Fcn/1

== system MGDC_COMPARACION/DC CONVERTER (RL) 1/Secundario  ==
  ref : Inport
  Vo : Inport  Port=2
  Constant3 : Constant  Value=10
  MATLAB Function1 : MATLAB Function  TreatAsAtomicUnit=on
  MATLAB Function2 : MATLAB Function  TreatAsAtomicUnit=on
  MATLAB Function3 : MATLAB Function  TreatAsAtomicUnit=on
  vs/accion : Outport
  wires:
  ref/1 -> MATLAB Function3/1(ref)
  Constant3/1 -> MATLAB Function2/2(N)
  MATLAB Function2/1(bin) -> MATLAB Function1/1(s)
  Vo/1 -> MATLAB Function3/2(V)
  MATLAB Function3/1(e) -> MATLAB Function2/1(e)
  MATLAB Function1/1(u) -> vs/accion/1

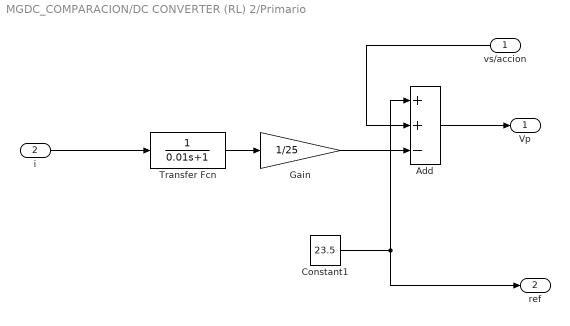
== system MGDC_COMPARACION/DC CONVERTER (RL) 2/Primario ==
  vs/accion : Inport
  i : Inport  Port=2
  Add : Sum  Inputs=++-
  Constant1 : Constant  Value=23.5
  Gain : Gain  Gain=1/25
  Transfer Fcn : TransferFcn  Denominator=[0.01 1]
  Vp : Outport
  ref : Outport  Port=2
  wires:
  vs/accion/1 -> Add/2
  Transfer Fcn/1 -> Gain/1
  Add/1 -> Vp/1
  Constant1/1 -> Add/1, ref/1
  Gain/1 -> Add/3
  i/1 -> Transfer Fcn/1

== system MGDC_COMPARACION/DC CONVERTER (RL) 2/Secundario  ==
  ref : Inport
  Vo : Inport  Port=2
  Constant3 : Constant  Value=10
  MATLAB Function1 : MATLAB Function  TreatAsAtomicUnit=on
  MATLAB Function2 : MATLAB Function  TreatAsAtomicUnit=on
  MATLAB Function3 : MATLAB Function  TreatAsAtomicUnit=on
  vs/accion : Outport
  wires:
  ref/1 -> MATLAB Function3/1(ref)
  Constant3/1 -> MATLAB Function2/2(N)
  MATLAB Function2/1(bin) -> MATLAB Function1/1(s)
  Vo/1 -> MATLAB Function3/2(V)
  MATLAB Function3/1(e) -> MATLAB Function2/1(e)
  MATLAB Function1/1(u) -> vs/accion/1

== system MGDC_COMPARACION/DC CONVERTER (RL) 3/Primario ==
  vs/accion : Inport
  i : Inport  Port=2
  Add : Sum  Inputs=++-
  Constant1 : Constant  Value=23.5
  Gain : Gain  Gain=1/50
  Transfer Fcn : TransferFcn  Denominator=[0.01 1]
  Vp : Outport
  ref : Outport  Port=2
  wires:
  vs/accion/1 -> Add/2
  Transfer Fcn/1 -> Gain/1
  Add/1 -> Vp/1
  Constant1/1 -> Add/1, ref/1
  Gain/1 -> Add/3
  i/1 -> Transfer Fcn/1

== system MGDC_COMPARACION/DC CONVERTER (RL) 3/Secundario  ==
  ref : Inport
  Vo : Inport  Port=2
  Constant3 : Constant  Value=10
  MATLAB Function1 : MATLAB Function  TreatAsAtomicUnit=on
  MATLAB Function2 : MATLAB Function  TreatAsAtomicUnit=on
  MATLAB Function3 : MATLAB Function  TreatAsAtomicUnit=on
  vs/accion : Outport
  wires:
  ref/1 -> MATLAB Function3/1(ref)
  Constant3/1 -> MATLAB Function2/2(N)
  MATLAB Function2/1(bin) -> MATLAB Function1/1(s)
  Vo/1 -> MATLAB Function3/2(V)
  MATLAB Function3/1(e) -> MATLAB Function2/1(e)
  MATLAB Function1/1(u) -> vs/accion/1
